simulink model "Step_2"  (Simulink 7.2)
settings: Solver=ode23t  StartTime=0.0  StopTime=inf  FixedStep=0.1  MaxStep=1  RelTol=1e-3
model workspace (MAT data in the model file):
  k = 0.01
  h0 = 1
  r2h : num (value not decoded)
PreLoadFcn:
  | bdclose all
libraries: simulink x5, sfWorkshop_libs x2, gaugeslibv2 x1
settings Model: Creator=wcampbel  LastModifiedBy=wcampbel
settings OptimizationCC: InitFltsAndDblsToZero=on

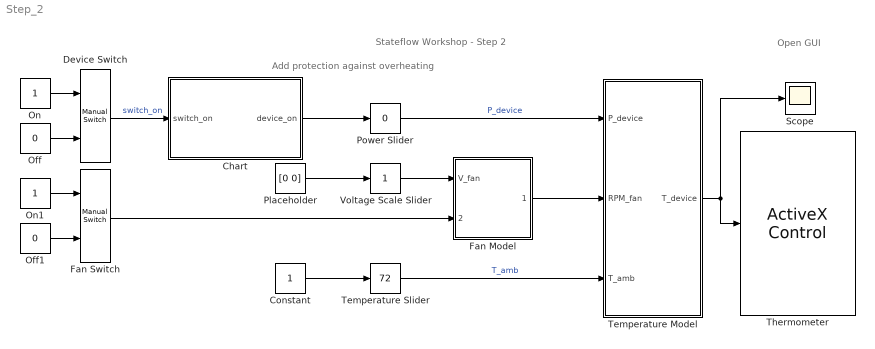
== system Step_2 ==
  note: Stateflow Workshop - Step 2
  note: Add protection against overheating
  note: Open GUI
  Chart : Stateflow chart
  Constant : Constant  OutDataType=sfix(16)  OutScaling=2^0
  Device Switch : simulink/Signal Routing/Manual Switch  SystemSampleTime=-1  sw=0  action=0  varsize=off
  Fan Model : Subsystem  BlockChoice=Advanced
      settings: TemplateBlock=sfWorkshop_libs/Fan Model  MemberBlocks=Advanced,Simple
  Fan Switch : simulink/Signal Routing/Manual Switch  SystemSampleTime=-1  sw=1  action=0  varsize=off
  Off : Constant  Value=0  OutDataType=sfix(16)  OutScaling=2^0
  Off1 : Constant  Value=0  OutDataType=sfix(16)  OutScaling=2^0
  On : Constant  OutDataType=sfix(16)  OutScaling=2^0
  On1 : Constant  OutDataType=sfix(16)  OutScaling=2^0
  Placeholder : Constant  Value=[0 0]  OutDataType=sfix(16)  OutScaling=2^0
  Power Slider : simulink/Math Operations/Slider Gain  SystemSampleTime=-1  low=0  gain=0  high=400
  Scope : Scope
  Temperature Model : Subsystem  BlockChoice=(Pace Control)
      settings: TemplateBlock=sfWorkshop_libs/Temperature Model  MemberBlocks=(No Pace Control),(Pace Control)
  Temperature Slider : simulink/Math Operations/Slider Gain  SystemSampleTime=-1  low=0  gain=72  high=125
  Thermometer : gaugeslibv2/ActiveX Control  Tag=000  progid=mwslider.sliderctrl.1  connect=input  input=Value  init=hActx.configuration='Slider\Thermometer'; hActx.MouseControl = 'NoMouseControl';  inblock=on  border=on  updateParam=0
  Voltage Scale Slider : simulink/Math Operations/Slider Gain  SystemSampleTime=-1  low=0  gain=1  high=2
  wires:
  On/1 -> Device Switch/1
  Off/1 -> Device Switch/2
  Constant/1 -> Temperature Slider/1
  Device Switch/1 -> Chart/1(switch_on)  "switch_on"
  Placeholder/1 -> Voltage Scale Slider/1
  Temperature Model/1(T_device) -> Scope/1, Thermometer/1
  Power Slider/1 -> Temperature Model/1(P_device)  "P_device"
  Temperature Slider/1 -> Temperature Model/3(T_amb)  "T_amb"
  Fan Model/1(RPM_fan) -> Temperature Model/2(RPM_fan)
  Voltage Scale Slider/1 -> Fan Model/1(V_fan)
  On1/1 -> Fan Switch/1
  Off1/1 -> Fan Switch/2
  Fan Switch/1 -> Fan Model/2(Override)
  Chart/1(device_on) -> Power Slider/1

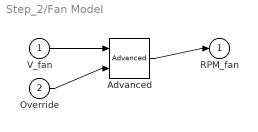
== system Step_2/Fan Model ==
  V_fan : Inport
  Override : Inport  Port=2
  Advanced : sfWorkshop_libs/Advanced  SystemSampleTime=-1
  RPM_fan : Outport
  wires:
  Advanced/1 -> RPM_fan/1
  Override/1 -> Advanced/2
  V_fan/1 -> Advanced/1

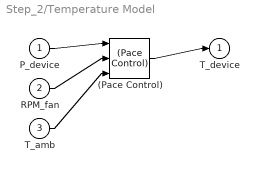
== system Step_2/Temperature Model ==
  P_device : Inport
  RPM_fan : Inport  Port=2
  T_amb : Inport  Port=3
  (Pace Control) : sfWorkshop_libs/(Pace Control)  SystemSampleTime=-1
  T_device : Outport
  wires:
  P_device/1 -> (Pace Control)/1
  RPM_fan/1 -> (Pace Control)/2
  T_amb/1 -> (Pace Control)/3
  (Pace Control)/1 -> T_device/1

== stateflow chart Chart ==
  state DeviceOn
    entry: device_on = 1;
  state DeviceOff
    entry: device_on = 0;
  DeviceOff -> DeviceOn : [switch_on]
  DeviceOn -> DeviceOff : [!switch_on]
  (default) -> DeviceOff
  data: device_on output double; switch_on input double
